simulink model "P1"  (R2020b)
settings: Solver=VariableStepAuto  StartTime=0.0  StopTime=10  RelTol=1e-3
settings Model: Creator=abdullah  LastModifiedBy=abdullah

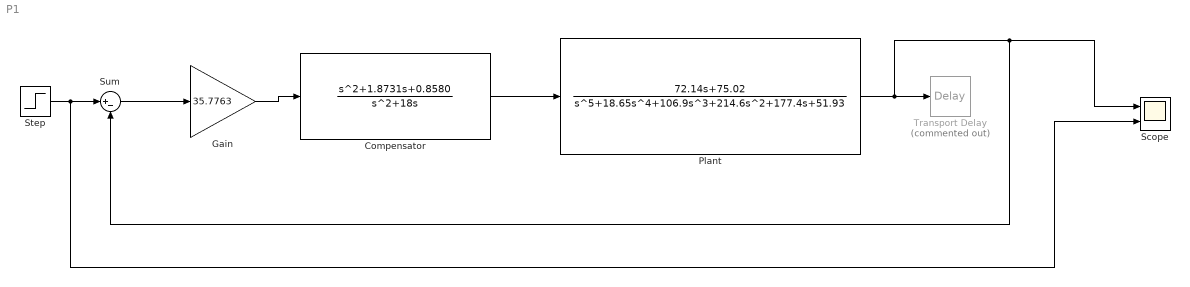
== system P1 ==
  Compensator : TransferFcn  Numerator=[1 1.8731 0.8580]  Denominator=[1 18 0]  ContinuousStateAttributes='Compensator'
  Gain : Gain  Gain=35.7763
  Plant : TransferFcn  Numerator=[72.14 75.02]  Denominator=[1 18.65 106.9 214.6 177.4 51.93]  ContinuousStateAttributes="\"Plant\""
  Scope : Scope  NumInputPorts=2
  Step : Step  SampleTime=0
  Sum : Sum  Inputs=|+-
  Transport Delay : TransportDelay  Commented=on  DelayTime=0.1
  wires:
  Sum/1 -> Gain/1
  Gain/1 -> Compensator/1
  Compensator/1 -> Plant/1
  Step/1 -> Scope/2, Sum/1
  Plant/1 -> Scope/1, Sum/2, Transport Delay/1
